simulink subsystem "Sub_LQR_Controller"  (R2021b)
settings: Solver=VariableStepAuto  StartTime=0.0  StopTime=10.0  RelTol=1e-3
undefined symbols (not defined in the file): K, Nbar
settings Model: Creator=Otonom  LastModifiedBy=Otonom

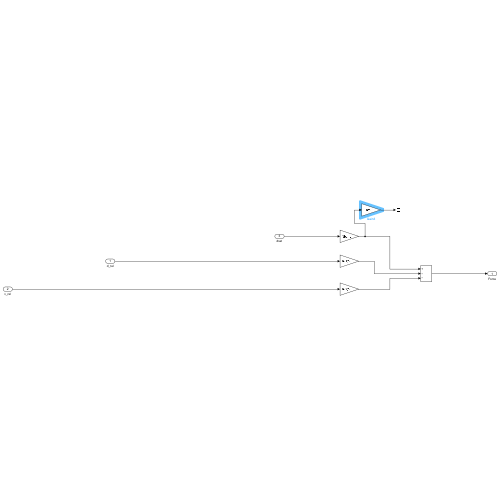
[thumbnail: Simulink's stored preview of the top-level diagram]
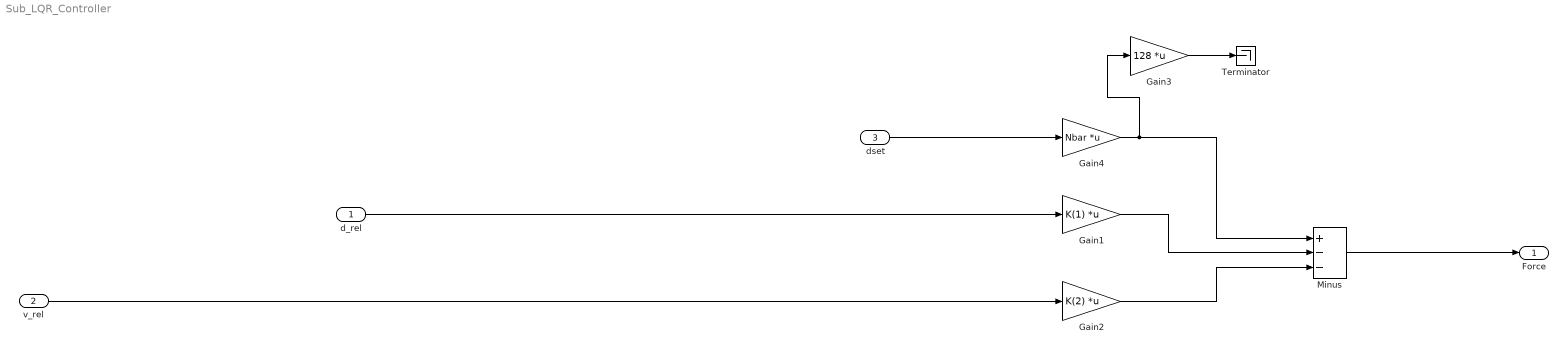
== system Sub_LQR_Controller ==
  d_rel : Inport
  v_rel : Inport  Port=2
  dset : Inport  Port=3
  Gain1 : Gain  Gain=K(1)  Multiplication=Matrix(K*u)
  Gain2 : Gain  Gain=K(2)  Multiplication=Matrix(K*u)
  Gain3 : Gain  Gain=128  Multiplication=Matrix(K*u)
  Gain4 : Gain  Gain=Nbar  Multiplication=Matrix(K*u)
  Minus : Sum  Inputs=+--
  Terminator : Terminator
  Force : Outport
  wires:
  dset/1 -> Gain4/1
  Gain1/1 -> Minus/2
  v_rel/1 -> Gain2/1
  Gain2/1 -> Minus/3
  Gain4/1 -> Gain3/1, Minus/1
  d_rel/1 -> Gain1/1
  Minus/1 -> Force/1
  Gain3/1 -> Terminator/1
